simulink model "LCW_a"  (Simulink 8.7)
settings: Solver=ode1  SolverMode=SingleTasking  StartTime=0.0  StopTime=500  FixedStep=0.001  RelTol=1e-3
(part 3 of 4)

== system LCW_a/Veh_1/ComplexVehicleModel/Body and Tires/body_kinematic_out_whl_lf2 ==
  In1 : Inport
  Bus Creator : BusCreator  Inputs=18
  Demux : Demux  Outputs=18
  Out1 : Outport
  wires:
  In1/1 -> Demux/1
  Demux/1 -> Bus Creator/1  "rot_whl"
  Demux/2 -> Bus Creator/2  "w_whl"
  Demux/3 -> Bus Creator/3  "z_whl_whl"
  Demux/4 -> Bus Creator/4  "yaw_whl"
  Demux/5 -> Bus Creator/5  "pitch_whl"
  Demux/6 -> Bus Creator/6  "roll_whl"
  Demux/7 -> Bus Creator/7  "vwx_whl"
  Demux/8 -> Bus Creator/8  "vwy_whl"
  Demux/9 -> Bus Creator/9  "vwz_whl"
  Demux/10 -> Bus Creator/10  "avwx_whl"
  Demux/11 -> Bus Creator/11  "avwy_whl"
  Demux/12 -> Bus Creator/12  "avwz_whl"
  Demux/13 -> Bus Creator/13  "dzdx_whl"
  Demux/14 -> Bus Creator/14  "dzdy_whl"
  Demux/15 -> Bus Creator/15  "xgnd_whl"
  Demux/16 -> Bus Creator/16  "ygnd_whl"
  Demux/17 -> Bus Creator/17  "zgnd_whl"
  Demux/18 -> Bus Creator/18  "mux_whl"
  Bus Creator/1 -> Out1/1  "bodykin_whl_out"

== system LCW_a/Veh_1/ComplexVehicleModel/Body and Tires/body_kinematic_out_whl_lf3 ==
  In1 : Inport
  Bus Creator : BusCreator  Inputs=18
  Demux : Demux  Outputs=18
  Out1 : Outport
  wires:
  Bus Creator/1 -> Out1/1  "bodykin_whl_out"
  Demux/18 -> Bus Creator/18  "mux_whl"
  Demux/17 -> Bus Creator/17  "zgnd_whl"
  Demux/16 -> Bus Creator/16  "ygnd_whl"
  Demux/15 -> Bus Creator/15  "xgnd_whl"
  Demux/14 -> Bus Creator/14  "dzdy_whl"
  Demux/13 -> Bus Creator/13  "dzdx_whl"
  Demux/12 -> Bus Creator/12  "avwz_whl"
  Demux/11 -> Bus Creator/11  "avwy_whl"
  Demux/10 -> Bus Creator/10  "avwx_whl"
  Demux/9 -> Bus Creator/9  "vwz_whl"
  Demux/8 -> Bus Creator/8  "vwy_whl"
  Demux/7 -> Bus Creator/7  "vwx_whl"
  Demux/6 -> Bus Creator/6  "roll_whl"
  Demux/5 -> Bus Creator/5  "pitch_whl"
  Demux/4 -> Bus Creator/4  "yaw_whl"
  Demux/3 -> Bus Creator/3  "z_whl_whl"
  Demux/2 -> Bus Creator/2  "w_whl"
  Demux/1 -> Bus Creator/1  "rot_whl"
  In1/1 -> Demux/1

== system LCW_a/Veh_1/ComplexVehicleModel/Brake/Brake States ==
  In1 : Inport
  Bus Creator : BusCreator  Inputs=26
  Demux : Demux  Outputs=26
  Out1 : Outport
  wires:
  In1/1 -> Demux/1
  Demux/1 -> Bus Creator/1  "q0"
  Demux/2 -> Bus Creator/2  "q1"
  Demux/3 -> Bus Creator/3  "q2"
  Demux/4 -> Bus Creator/4  "q3"
  Demux/5 -> Bus Creator/5  "q4"
  Demux/6 -> Bus Creator/6  "q5"
  Demux/7 -> Bus Creator/7  "q6"
  Demux/8 -> Bus Creator/8  "q7"
  Demux/9 -> Bus Creator/9  "q8"
  Demux/10 -> Bus Creator/10  "q9"
  Demux/11 -> Bus Creator/11  "q10"
  Demux/12 -> Bus Creator/12  "q11"
  Demux/13 -> Bus Creator/13  "q12"
  Demux/14 -> Bus Creator/14  "u0"
  Demux/15 -> Bus Creator/15  "u1"
  Demux/16 -> Bus Creator/16  "u2"
  Bus Creator/1 -> Out1/1  "BrakeStates"
  Demux/17 -> Bus Creator/17  "u3"
  Demux/18 -> Bus Creator/18  "u4"
  Demux/19 -> Bus Creator/19  "u5"
  Demux/20 -> Bus Creator/20  "u6"
  Demux/21 -> Bus Creator/21  "u7"
  Demux/22 -> Bus Creator/22  "u8"
  Demux/23 -> Bus Creator/23  "u9"
  Demux/24 -> Bus Creator/24  "u10"
  Demux/25 -> Bus Creator/25  "u11"
  Demux/26 -> Bus Creator/26  "u12"

== system LCW_a/Veh_1/ComplexVehicleModel/Brake/SteerStates1 ==
  In1 : Inport
  Bus Creator : BusCreator  Inputs=22
  Demux : Demux  Outputs=22
  Out1 : Outport
  wires:
  Demux/22 -> Bus Creator/22  "turn_off"
  Demux/21 -> Bus Creator/21  "brake"
  Demux/20 -> Bus Creator/20  "trot_brk_rr"
  Demux/19 -> Bus Creator/19  "trot_brk_lr"
  Demux/18 -> Bus Creator/18  "trot_brk_rf"
  Demux/17 -> Bus Creator/17  "trot_brk_lf"
  Bus Creator/1 -> Out1/1  "BrakeOutput"
  Demux/16 -> Bus Creator/16  "mu_us_brk_rr"
  Demux/15 -> Bus Creator/15  "mu_us_brk_lr"
  Demux/14 -> Bus Creator/14  "mu_us_brk_rf"
  Demux/13 -> Bus Creator/13  "mu_us_brk_lf"
  Demux/12 -> Bus Creator/12  "fm_brk_rr"
  Demux/11 -> Bus Creator/11  "fm_brk_lr"
  Demux/10 -> Bus Creator/10  "fm_brk_rf"
  Demux/9 -> Bus Creator/9  "fm_brk_lf"
  Demux/8 -> Bus Creator/8  "pbkch_brk_rr"
  Demux/7 -> Bus Creator/7  "pbkch_brk_lr"
  Demux/6 -> Bus Creator/6  "pbkch_brk_rf"
  Demux/5 -> Bus Creator/5  "pbkch_brk_lf"
  Demux/4 -> Bus Creator/4  "fbk_out_brk"
  Demux/3 -> Bus Creator/3  "fbk_in_brk"
  Demux/2 -> Bus Creator/2  "fbk_pedal"
  Demux/1 -> Bus Creator/1  "pbk_con_brk"
  In1/1 -> Demux/1

== system LCW_a/Veh_1/ComplexVehicleModel/Powertrain/PowertrainOut ==
  In1 : Inport
  Bus Creator : BusCreator  Inputs=36
  Demux : Demux  Outputs=36
  Out1 : Outport
  wires:
  Bus Creator/1 -> Out1/1  "PowertrainOut"
  In1/1 -> Demux/1
  Demux/1 -> Bus Creator/1  "aa_eng"
  Demux/2 -> Bus Creator/2  "av_eng"
  Demux/3 -> Bus Creator/3  "av_eng_update"
  Demux/4 -> Bus Creator/4  "av_tc"
  Demux/5 -> Bus Creator/5  "fuel"
  Demux/6 -> Bus Creator/6  "iw_eff_pt_lf"
  Demux/7 -> Bus Creator/7  "iw_eff_pt_rf"
  Demux/8 -> Bus Creator/8  "iw_eff_pt_lr"
  Demux/9 -> Bus Creator/9  "iw_eff_pt_rr"
  Demux/10 -> Bus Creator/10  "my_drv_lf"
  Demux/11 -> Bus Creator/11  "my_drv_rf"
  Demux/12 -> Bus Creator/12  "my_drv_lr"
  Demux/13 -> Bus Creator/13  "my_drv_rr"
  Demux/14 -> Bus Creator/14  "pt_thr_eng"
  Demux/15 -> Bus Creator/15  "pt_throttle"
  Demux/16 -> Bus Creator/16  "pt_modetran"
  Demux/17 -> Bus Creator/17  "pt_rottrans"
  Demux/18 -> Bus Creator/18  "pt_m_engout"
  Demux/19 -> Bus Creator/19  "pt_m_eng_in"
  Demux/20 -> Bus Creator/20  "pt_gearauto"
  Demux/21 -> Bus Creator/21  "pt_gear_status"
  Demux/22 -> Bus Creator/22  "pt_gear_man"
  Demux/23 -> Bus Creator/23  "rot_eng_update"
  Demux/24 -> Bus Creator/24  "rot_tc"
  Demux/25 -> Bus Creator/25  "pt_av_trans"
  Demux/26 -> Bus Creator/26  "pt_m_tc"
  Demux/27 -> Bus Creator/27  "pt_m_trans"
  Demux/28 -> Bus Creator/28  "pt_pwrengin"
  Demux/29 -> Bus Creator/29  "pt_pwrengo"
  Demux/30 -> Bus Creator/30  "pt_pwrtrans"
  Demux/31 -> Bus Creator/31  "pt_pwrwheel"
  Demux/32 -> Bus Creator/32  "pt_pwr_tc"
  Demux/33 -> Bus Creator/33  "pt_clutch"
  Demux/34 -> Bus Creator/34  "pt_k_tc"
  Demux/35 -> Bus Creator/35  "pt_r_av_tc"
  Demux/36 -> Bus Creator/36  "pt_r_m_tc"

== system LCW_a/Veh_1/ComplexVehicleModel/Powertrain/PowertrainStates ==
  In1 : Inport
  Bus Creator : BusCreator  Inputs=38
  Demux : Demux  Outputs=38
  Out1 : Outport
  wires:
  In1/1 -> Demux/1
  Bus Creator/1 -> Out1/1  "PowertrainStates"
  Demux/1 -> Bus Creator/1  "q0"
  Demux/2 -> Bus Creator/2  "q1"
  Demux/3 -> Bus Creator/3  "q2"
  Demux/4 -> Bus Creator/4  "q3"
  Demux/5 -> Bus Creator/5  "q4"
  Demux/6 -> Bus Creator/6  "q5"
  Demux/7 -> Bus Creator/7  "q6"
  Demux/8 -> Bus Creator/8  "q7"
  Demux/9 -> Bus Creator/9  "q8"
  Demux/10 -> Bus Creator/10  "q9"
  Demux/11 -> Bus Creator/11  "q10"
  Demux/12 -> Bus Creator/12  "q11"
  Demux/13 -> Bus Creator/13  "q12"
  Demux/14 -> Bus Creator/14  "q13"
  Demux/15 -> Bus Creator/15  "q14"
  Demux/16 -> Bus Creator/16  "q15"
  Demux/17 -> Bus Creator/17  "q16"
  Demux/18 -> Bus Creator/18  "q17"
  Demux/19 -> Bus Creator/19  "q18"
  Demux/20 -> Bus Creator/20  "u0"
  Demux/21 -> Bus Creator/21  "u1"
  Demux/22 -> Bus Creator/22  "u2"
  Demux/23 -> Bus Creator/23  "u3"
  Demux/24 -> Bus Creator/24  "u4"
  Demux/25 -> Bus Creator/25  "u5"
  Demux/26 -> Bus Creator/26  "u6"
  Demux/27 -> Bus Creator/27  "u7"
  Demux/28 -> Bus Creator/28  "u8"
  Demux/29 -> Bus Creator/29  "u9"
  Demux/30 -> Bus Creator/30  "u10"
  Demux/31 -> Bus Creator/31  "u11"
  Demux/32 -> Bus Creator/32  "u12"
  Demux/33 -> Bus Creator/33  "u13"
  Demux/34 -> Bus Creator/34  "u14"
  Demux/35 -> Bus Creator/35  "u15"
  Demux/36 -> Bus Creator/36  "u16"
  Demux/37 -> Bus Creator/37  "u17"
  Demux/38 -> Bus Creator/38  "u18"

== system LCW_a/Veh_1/ComplexVehicleModel/Steer/SteerForces ==
  In1 : Inport
  Bus Creator : BusCreator  Inputs=32
  Demux : Demux  Outputs=32
  Out1 : Outport
  wires:
  Bus Creator/1 -> Out1/1  "Steer_Forces"
  Demux/26 -> Bus Creator/26  "steer_f_hys_2"
  Demux/25 -> Bus Creator/25  "steer_f_hys_1"
  Demux/24 -> Bus Creator/24  "steer_mkp_in_4"
  Demux/23 -> Bus Creator/23  "steer_mkp_in_3"
  Demux/22 -> Bus Creator/22  "steer_mkp_in_2"
  Demux/21 -> Bus Creator/21  "steer_mkp_in_1"
  Demux/20 -> Bus Creator/20  "steer_gear_dam_f_2"
  Demux/19 -> Bus Creator/19  "steer_boost_f_2"
  Demux/18 -> Bus Creator/18  "steer_gear_dam_t_2"
  Demux/17 -> Bus Creator/17  "steer_boost_t_2"
  Demux/16 -> Bus Creator/16  "steer_gear_dam_f_1"
  Demux/15 -> Bus Creator/15  "steer_boost_f_1"
  Demux/14 -> Bus Creator/14  "steer_gear_dam_t_1"
  Demux/13 -> Bus Creator/13  "steer_boost_t_1"
  Demux/12 -> Bus Creator/12  "steer_col_fric_t3"
  Demux/11 -> Bus Creator/11  "steer_col_dam_t3"
  Demux/10 -> Bus Creator/10  "steer_col_fric_t2"
  Demux/9 -> Bus Creator/9  "steer_col_dam_t2"
  Demux/8 -> Bus Creator/8  "steer_t_in1"
  Demux/7 -> Bus Creator/7  "steer_tbar_t1"
  Demux/6 -> Bus Creator/6  "steer_col_fric_t1"
  Demux/5 -> Bus Creator/5  "steer_col_dam_t1"
  Demux/4 -> Bus Creator/4  "steer_tbar_t"
  Demux/3 -> Bus Creator/3  "steer_col_fric_t"
  Demux/2 -> Bus Creator/2  "steer_col_dam_t"
  Demux/1 -> Bus Creator/1  "steer_t_in"
  In1/1 -> Demux/1
  Demux/27 -> Bus Creator/27  "steer_f_hys_3"
  Demux/28 -> Bus Creator/28  "steer_f_hys_4"
  Demux/29 -> Bus Creator/29  "m_kp_str_1"
  Demux/30 -> Bus Creator/30  "m_kp_str_2"
  Demux/31 -> Bus Creator/31  "m_kp_str_3"
  Demux/32 -> Bus Creator/32  "m_kp_str_4"

== system LCW_a/Veh_1/ComplexVehicleModel/Steer/SteerKinemateics ==
  In1 : Inport
  Bus Creator : BusCreator  Inputs=9
  Demux : Demux  Outputs=[4 1 1 1 1 4 4 4 2]
  Out1 : Outport
  wires:
  Bus Creator/1 -> Out1/1  "Steer_Kinematics"
  Demux/8 -> Bus Creator/8  "k_str"
  Demux/7 -> Bus Creator/7  "c_str"
  Demux/6 -> Bus Creator/6  "steer_str"
  Demux/5 -> Bus Creator/5  "str_sus_r"
  Demux/4 -> Bus Creator/4  "str_sus_f"
  Demux/3 -> Bus Creator/3  "strav_sw"
  Demux/2 -> Bus Creator/2  "drstr"
  Demux/1 -> Bus Creator/1  "str_whl_opt"
  In1/1 -> Demux/1
  Demux/9 -> Bus Creator/9  "strswr"

== system LCW_a/Veh_1/ComplexVehicleModel/Steer/SteerStates ==
  In1 : Inport
  Bus Creator : BusCreator  Inputs=26
  Demux : Demux  Outputs=26
  Out1 : Outport
  wires:
  In1/1 -> Demux/1
  Demux/1 -> Bus Creator/1  "q0"
  Demux/2 -> Bus Creator/2  "q1"
  Demux/3 -> Bus Creator/3  "q2"
  Demux/4 -> Bus Creator/4  "q3"
  Demux/5 -> Bus Creator/5  "q4"
  Demux/6 -> Bus Creator/6  "q5"
  Demux/7 -> Bus Creator/7  "q6"
  Demux/8 -> Bus Creator/8  "q7"
  Demux/9 -> Bus Creator/9  "q8"
  Demux/10 -> Bus Creator/10  "q9"
  Demux/11 -> Bus Creator/11  "q10"
  Demux/12 -> Bus Creator/12  "q11"
  Demux/13 -> Bus Creator/13  "q12"
  Demux/14 -> Bus Creator/14  "u0"
  Demux/15 -> Bus Creator/15  "u1"
  Demux/16 -> Bus Creator/16  "u2"
  Bus Creator/1 -> Out1/1  "SteerStates"
  Demux/17 -> Bus Creator/17  "u3"
  Demux/18 -> Bus Creator/18  "u4"
  Demux/19 -> Bus Creator/19  "u5"
  Demux/20 -> Bus Creator/20  "u6"
  Demux/21 -> Bus Creator/21  "u7"
  Demux/22 -> Bus Creator/22  "u8"
  Demux/23 -> Bus Creator/23  "u9"
  Demux/24 -> Bus Creator/24  "u10"
  Demux/25 -> Bus Creator/25  "u11"
  Demux/26 -> Bus Creator/26  "u12"

== system LCW_a/Veh_1/ComplexVehicleModel/Steer/SteerToBody ==
  In1 : Inport
  Bus Creator : BusCreator  Inputs=7
  Demux : Demux  Outputs=[2 4 4 4 4 4 4]
  Out1 : Outport
  wires:
  In1/1 -> Demux/1
  Demux/1 -> Bus Creator/1  "strratio"
  Demux/2 -> Bus Creator/2  "strc_str"
  Demux/3 -> Bus Creator/3  "kppc_str"
  Demux/4 -> Bus Creator/4  "kprc_str"
  Demux/5 -> Bus Creator/5  "rotd_kp_dr_str"
  Demux/6 -> Bus Creator/6  "rotd_kp_susp_str"
  Demux/7 -> Bus Creator/7  "gear_rotd_susp_str"
  Bus Creator/1 -> Out1/1  "Steer2Body"

== system LCW_a/Veh_1/ComplexVehicleModel/Suspensions/SupensionsStates ==
  In1 : Inport
  Bus Creator : BusCreator  Inputs=32
  Demux : Demux  Outputs=32
  Out1 : Outport
  wires:
  In1/1 -> Demux/1
  Demux/1 -> Bus Creator/1  "q0"
  Demux/2 -> Bus Creator/2  "q1"
  Demux/3 -> Bus Creator/3  "q2"
  Demux/4 -> Bus Creator/4  "q3"
  Demux/5 -> Bus Creator/5  "q4"
  Demux/6 -> Bus Creator/6  "q5"
  Demux/7 -> Bus Creator/7  "q6"
  Demux/8 -> Bus Creator/8  "q7"
  Demux/9 -> Bus Creator/9  "q8"
  Demux/10 -> Bus Creator/10  "q9"
  Demux/11 -> Bus Creator/11  "q10"
  Demux/12 -> Bus Creator/12  "q11"
  Demux/13 -> Bus Creator/13  "q12"
  Demux/14 -> Bus Creator/14  "q13"
  Demux/15 -> Bus Creator/15  "q14"
  Demux/16 -> Bus Creator/16  "q15"
  Bus Creator/1 -> Out1/1  "Suspensions States"
  Demux/17 -> Bus Creator/17  "u0"
  Demux/18 -> Bus Creator/18  "u1"
  Demux/19 -> Bus Creator/19  "u2"
  Demux/20 -> Bus Creator/20  "u3"
  Demux/21 -> Bus Creator/21  "u4"
  Demux/22 -> Bus Creator/22  "u5"
  Demux/23 -> Bus Creator/23  "u6"
  Demux/24 -> Bus Creator/24  "u7"
  Demux/25 -> Bus Creator/25  "u8"
  Demux/26 -> Bus Creator/26  "u9"
  Demux/27 -> Bus Creator/27  "u10"
  Demux/28 -> Bus Creator/28  "u11"
  Demux/29 -> Bus Creator/29  "u12"
  Demux/30 -> Bus Creator/30  "u13"
  Demux/31 -> Bus Creator/31  "u14"
  Demux/32 -> Bus Creator/32  "u15"

== system LCW_a/Veh_1/ComplexVehicleModel/Suspensions/SuspensionForces ==
  In1 : Inport
  Bus Creator : BusCreator  Inputs=18
  Demux : Demux  Outputs=18
  Out1 : Outport
  wires:
  Bus Creator/1 -> Out1/1  "SuspensionForces"
  In1/1 -> Demux/1
  Demux/1 -> Bus Creator/1  "spring_f_r1"
  Demux/2 -> Bus Creator/2  "spring_f_l1"
  Demux/3 -> Bus Creator/3  "spring_f_r2"
  Demux/4 -> Bus Creator/4  "spring_f_l2"
  Demux/5 -> Bus Creator/5  "jounce_stop_f_r1"
  Demux/6 -> Bus Creator/6  "reound_stop_f_r1"
  Demux/7 -> Bus Creator/7  "jounce_stop_f_l1"
  Demux/8 -> Bus Creator/8  "reound_stop_f_l1"
  Demux/9 -> Bus Creator/9  "jounce_stop_f_r2"
  Demux/10 -> Bus Creator/10  "reound_stop_f_r2"
  Demux/11 -> Bus Creator/11  "jounce_stop_f_l2"
  Demux/12 -> Bus Creator/12  "reound_stop_f_l2"
  Demux/13 -> Bus Creator/13  "damper_l1"
  Demux/14 -> Bus Creator/14  "damper_r1"
  Demux/15 -> Bus Creator/15  "damper_l2"
  Demux/16 -> Bus Creator/16  "damper_r2"
  Demux/17 -> Bus Creator/17  "maux_f"
  Demux/18 -> Bus Creator/18  "maux_r"

== system LCW_a/Veh_1/ComplexVehicleModel/Suspensions/SuspensionKinematics ==
  In1 : Inport
  Bus Creator : BusCreator  Inputs=23
  Demux : Demux  Outputs=[4 4 4 4 4 4 4 4 4 4 4 4 4 4 4 4 4 4 4 4 4 4 4]
  Out1 : Outport
  wires:
  Demux/23 -> Bus Creator/23  "fs_ext_susp"
  Demux/22 -> Bus Creator/22  "fs_susp"
  Demux/21 -> Bus Creator/21  "cmp_s_susp"
  Demux/20 -> Bus Creator/20  "cmprst_susp"
  Demux/19 -> Bus Creator/19  "cmprd_susp"
  Demux/18 -> Bus Creator/18  "cmpjst_susp"
  Demux/17 -> Bus Creator/17  "dcam_con_susp"
  Bus Creator/1 -> Out1/1  "SuspensionsKinematiocs"
  Demux/16 -> Bus Creator/16  "divedd_susp"
  Demux/15 -> Bus Creator/15  "dived_susp"
  Demux/14 -> Bus Creator/14  "dive_susp"
  Demux/13 -> Bus Creator/13  "toedd_susp"
  Demux/12 -> Bus Creator/12  "toed_susp"
  Demux/11 -> Bus Creator/11  "toe_susp"
  Demux/10 -> Bus Creator/10  "camdd_susp"
  Demux/9 -> Bus Creator/9  "camd_susp"
  Demux/8 -> Bus Creator/8  "cam_con_susp"
  Demux/7 -> Bus Creator/7  "cam_susp"
  Demux/6 -> Bus Creator/6  "latdd_susp"
  Demux/5 -> Bus Creator/5  "latd_susp"
  Demux/4 -> Bus Creator/4  "lat_susp"
  Demux/3 -> Bus Creator/3  "xdd_susp"
  Demux/2 -> Bus Creator/2  "xd_susp"
  Demux/1 -> Bus Creator/1  "x_susp"
  In1/1 -> Demux/1

== system LCW_a/Veh_1/ComplexVehicleModel/Suspensions/SuspensionSteer ==
  In1 : Inport
  Bus Creator : BusCreator  Inputs=3
  Demux : Demux  Outputs=[4 4 4]
  Out1 : Outport
  wires:
  Bus Creator/1 -> Out1/1  "SuspensionSteer"
  Demux/3 -> Bus Creator/3  "sw_mz_susp"
  Demux/2 -> Bus Creator/2  "sw_fy_susp"
  Demux/1 -> Bus Creator/1  "sw_fx_susp"
  In1/1 -> Demux/1

== system LCW_a/Veh_1/DriverModel/Driver/Driver2Brake ==
  In1 : Inport
  Bus Creator : BusCreator  Inputs=1
  Demux : Demux  Outputs=1
  Out1 : Outport
  wires:
  In1/1 -> Demux/1
  Demux/1 -> Bus Creator/1  "pcon_bk"
  Bus Creator/1 -> Out1/1  "Driver2Brake"

== system LCW_a/Veh_1/DriverModel/Driver/Driver2Powertrain ==
  In1 : Inport
  Bus Creator : BusCreator  Inputs=3
  Demux : Demux  Outputs=3
  Out1 : Outport
  wires:
  Bus Creator/1 -> Out1/1  "Driver2Powertrain"
  Demux/1 -> Bus Creator/1  "throttle"
  In1/1 -> Demux/1
  Demux/2 -> Bus Creator/2  "modetr"
  Demux/3 -> Bus Creator/3  "geartr"

== system LCW_a/Veh_1/DriverModel/Driver/Driver2Steer ==
  In1 : Inport
  Bus Creator : BusCreator  Inputs=1
  Demux : Demux  Outputs=1
  Out1 : Outport
  wires:
  In1/1 -> Demux/1
  Demux/1 -> Bus Creator/1  "drstr_drv"
  Bus Creator/1 -> Out1/1  "Driver2Steer"

== system LCW_a/Veh_1/DriverModel/Driver/DriverStates ==
  In1 : Inport
  Bus Creator : BusCreator  Inputs=4
  Demux : Demux
  Out1 : Outport
  wires:
  Bus Creator/1 -> Out1/1  "DriverStates"
  Demux/4 -> Bus Creator/4  "my_sc_r"
  Demux/3 -> Bus Creator/3  "my_sc_f"
  Demux/2 -> Bus Creator/2  "verr_drv"
  Demux/1 -> Bus Creator/1  "iverr_drv"
  In1/1 -> Demux/1

== system LCW_a/Veh_1_1/ComplexVehicleModel/Aerodynamics/Chassis States ==
  In1 : Inport
  Bus Creator : BusCreator  Inputs=12
  Demux : Demux  Outputs=12
  Out1 : Outport
  wires:
  In1/1 -> Demux/1
  Demux/1 -> Bus Creator/1  "beta_air"
  Demux/2 -> Bus Creator/2  "pitch_air"
  Demux/3 -> Bus Creator/3  "yawwind_air"
  Demux/4 -> Bus Creator/4  "v_air"
  Demux/5 -> Bus Creator/5  "vwind_air"
  Demux/6 -> Bus Creator/6  "z_air"
  Demux/7 -> Bus Creator/7  "fx_air"
  Demux/8 -> Bus Creator/8  "fy_air"
  Demux/9 -> Bus Creator/9  "fz_air"
  Demux/10 -> Bus Creator/10  "mx_air"
  Demux/11 -> Bus Creator/11  "my_air"
  Demux/12 -> Bus Creator/12  "mz_air"
  Bus Creator/1 -> Out1/1  "Aerodynamics_States"

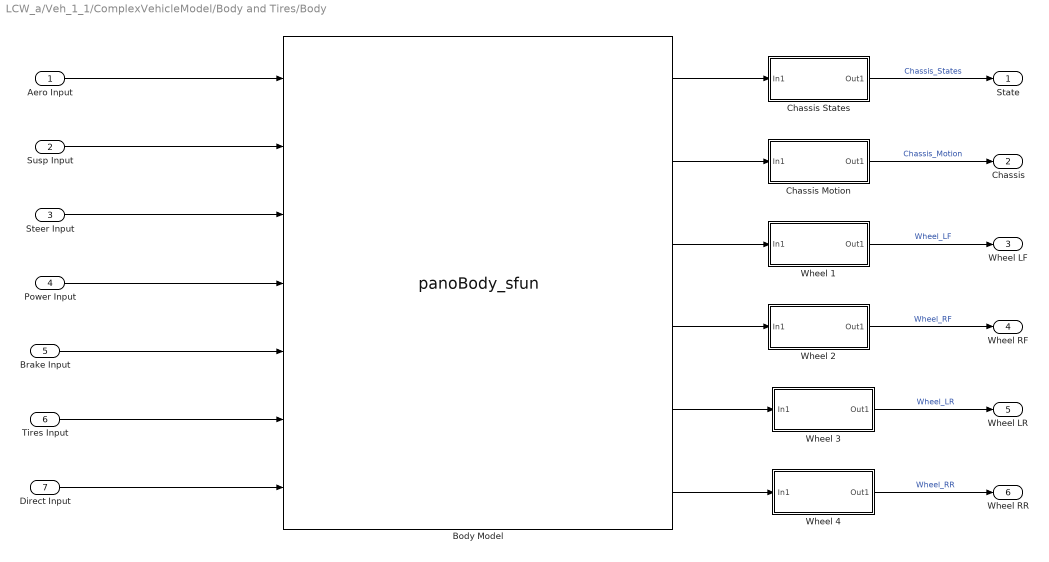
== system LCW_a/Veh_1_1/ComplexVehicleModel/Body and Tires/Body ==
  Aero Input : Inport
  Susp Input : Inport  Port=2
  Steer Input : Inport  Port=3
  Power Input : Inport  Port=4
  Brake Input : Inport  Port=5
  Tires Input : Inport  Port=6
  Direct Input : Inport  Port=7
  Body Model : S-Function  FunctionName=panoBody_sfun  Parameters='65ff4a6f-e423-428f-b9f1-c5e17da2fbba'  SFunctionDeploymentMode=off  EnableBusSupport=off
  Chassis Motion : Subsystem
  Chassis States : Subsystem
  Wheel 1 : Subsystem
  Wheel 2 : Subsystem
  Wheel 3 : Subsystem
  Wheel 4 : Subsystem
  State : Outport
  Chassis : Outport  Port=2
  Wheel LF : Outport  Port=3
  Wheel RF : Outport  Port=4
  Wheel LR : Outport  Port=5
  Wheel RR : Outport  Port=6
  wires:
  Direct Input/1 -> Body Model/7
  Body Model/2 -> Chassis Motion/1(In1)
  Chassis Motion/1(Out1) -> Chassis/1  "Chassis_Motion"
  Body Model/1 -> Chassis States/1(In1)
  Chassis States/1(Out1) -> State/1  "Chassis_States"
  Body Model/3 -> Wheel 1/1(In1)
  Wheel 1/1(Out1) -> Wheel LF/1  "Wheel_LF"
  Body Model/4 -> Wheel 2/1(In1)
  Body Model/5 -> Wheel 3/1(In1)
  Body Model/6 -> Wheel 4/1(In1)
  Wheel 3/1(Out1) -> Wheel LR/1  "Wheel_LR"
  Wheel 4/1(Out1) -> Wheel RR/1  "Wheel_RR"
  Wheel 2/1(Out1) -> Wheel RF/1  "Wheel_RF"
  Tires Input/1 -> Body Model/6
  Power Input/1 -> Body Model/4
  Brake Input/1 -> Body Model/5
  Steer Input/1 -> Body Model/3
  Susp Input/1 -> Body Model/2
  Aero Input/1 -> Body Model/1

== system LCW_a/Veh_1_1/ComplexVehicleModel/Body and Tires/Tires ==
  Wheel LF : Inport
  Wheel RF : Inport  Port=2
  Wheel LR : Inport  Port=3
  Wheel RR : Inport  Port=4
  Tires Force  2 : Subsystem
  "Tires Force 1 " : Subsystem
  Tires Force 3 : Subsystem
  Tires Force 4 : Subsystem
  Tires Force Ground : Subsystem
  Tires Model : S-Function  FunctionName=panoTire_sfun  Parameters='65ff4a6f-e423-428f-b9f1-c5e17da2fbba'  SFunctionDeploymentMode=off  EnableBusSupport=off
  TiresStates : Subsystem
  Tire States : Outport
  Tire LF : Outport  Port=2
  Tire RF : Outport  Port=3
  Tire LR : Outport  Port=4
  Tire RR : Outport  Port=5
  Tire Force Ground : Outport  Port=6
  wires:
  Tires Model/6 -> Tires Force Ground/1(In1)
  Tires Force Ground/1(Out1) -> Tire Force Ground/1  "Tire_Forces_GND"
  Wheel LF/1 -> Tires Model/1
  Wheel RF/1 -> Tires Model/2
  Wheel LR/1 -> Tires Model/3
  Wheel RR/1 -> Tires Model/4
  Tires Model/1 -> TiresStates/1(In1)
  TiresStates/1(Out1) -> Tire States/1  "Tires_States"
  Tires Model/2 -> "Tires Force 1 "/1(In1)
  "Tires Force 1 "/1(Out1) -> Tire LF/1  "Tire_Forces_LF"
  Tires Model/5 -> Tires Force 4/1(In1)
  Tires Model/4 -> Tires Force 3/1(In1)
  Tires Model/3 -> Tires Force  2/1(In1)
  Tires Force 3/1(Out1) -> Tire LR/1  "Tire_Forces_LR"
  Tires Force 4/1(Out1) -> Tire RR/1  "Tire_Forces_RR"
  Tires Force  2/1(Out1) -> Tire RF/1  "Tire_Forces_RF"

== system LCW_a/Veh_1_1/ComplexVehicleModel/Body and Tires/body_kinematic_out_whl_lf ==
  In1 : Inport
  Bus Creator : BusCreator  Inputs=18
  Demux : Demux  Outputs=18
  Out1 : Outport
  wires:
  In1/1 -> Demux/1
  Demux/1 -> Bus Creator/1  "rot_whl"
  Demux/2 -> Bus Creator/2  "w_whl"
  Demux/3 -> Bus Creator/3  "z_whl_whl"
  Demux/4 -> Bus Creator/4  "yaw_whl"
  Demux/5 -> Bus Creator/5  "pitch_whl"
  Demux/6 -> Bus Creator/6  "roll_whl"
  Demux/7 -> Bus Creator/7  "vwx_whl"
  Demux/8 -> Bus Creator/8  "vwy_whl"
  Demux/9 -> Bus Creator/9  "vwz_whl"
  Demux/10 -> Bus Creator/10  "avwx_whl"
  Demux/11 -> Bus Creator/11  "avwy_whl"
  Demux/12 -> Bus Creator/12  "avwz_whl"
  Demux/13 -> Bus Creator/13  "dzdx_whl"
  Demux/14 -> Bus Creator/14  "dzdy_whl"
  Demux/15 -> Bus Creator/15  "xgnd_whl"
  Demux/16 -> Bus Creator/16  "ygnd_whl"
  Demux/17 -> Bus Creator/17  "zgnd_whl"
  Demux/18 -> Bus Creator/18  "mux_whl"
  Bus Creator/1 -> Out1/1  "bodykin_whl_out"

== system LCW_a/Veh_1_1/ComplexVehicleModel/Body and Tires/body_kinematic_out_whl_lf1 ==
  In1 : Inport
  Bus Creator : BusCreator  Inputs=18
  Demux : Demux  Outputs=18
  Out1 : Outport
  wires:
  Bus Creator/1 -> Out1/1  "bodykin_whl_out"
  Demux/18 -> Bus Creator/18  "mux_whl"
  Demux/17 -> Bus Creator/17  "zgnd_whl"
  Demux/16 -> Bus Creator/16  "ygnd_whl"
  Demux/15 -> Bus Creator/15  "xgnd_whl"
  Demux/14 -> Bus Creator/14  "dzdy_whl"
  Demux/13 -> Bus Creator/13  "dzdx_whl"
  Demux/12 -> Bus Creator/12  "avwz_whl"
  Demux/11 -> Bus Creator/11  "avwy_whl"
  Demux/10 -> Bus Creator/10  "avwx_whl"
  Demux/9 -> Bus Creator/9  "vwz_whl"
  Demux/8 -> Bus Creator/8  "vwy_whl"
  Demux/7 -> Bus Creator/7  "vwx_whl"
  Demux/6 -> Bus Creator/6  "roll_whl"
  Demux/5 -> Bus Creator/5  "pitch_whl"
  Demux/4 -> Bus Creator/4  "yaw_whl"
  Demux/3 -> Bus Creator/3  "z_whl_whl"
  Demux/2 -> Bus Creator/2  "w_whl"
  Demux/1 -> Bus Creator/1  "rot_whl"
  In1/1 -> Demux/1

== system LCW_a/Veh_1_1/ComplexVehicleModel/Body and Tires/body_kinematic_out_whl_lf2 ==
  In1 : Inport
  Bus Creator : BusCreator  Inputs=18
  Demux : Demux  Outputs=18
  Out1 : Outport
  wires:
  In1/1 -> Demux/1
  Demux/1 -> Bus Creator/1  "rot_whl"
  Demux/2 -> Bus Creator/2  "w_whl"
  Demux/3 -> Bus Creator/3  "z_whl_whl"
  Demux/4 -> Bus Creator/4  "yaw_whl"
  Demux/5 -> Bus Creator/5  "pitch_whl"
  Demux/6 -> Bus Creator/6  "roll_whl"
  Demux/7 -> Bus Creator/7  "vwx_whl"
  Demux/8 -> Bus Creator/8  "vwy_whl"
  Demux/9 -> Bus Creator/9  "vwz_whl"
  Demux/10 -> Bus Creator/10  "avwx_whl"
  Demux/11 -> Bus Creator/11  "avwy_whl"
  Demux/12 -> Bus Creator/12  "avwz_whl"
  Demux/13 -> Bus Creator/13  "dzdx_whl"
  Demux/14 -> Bus Creator/14  "dzdy_whl"
  Demux/15 -> Bus Creator/15  "xgnd_whl"
  Demux/16 -> Bus Creator/16  "ygnd_whl"
  Demux/17 -> Bus Creator/17  "zgnd_whl"
  Demux/18 -> Bus Creator/18  "mux_whl"
  Bus Creator/1 -> Out1/1  "bodykin_whl_out"

== system LCW_a/Veh_1_1/ComplexVehicleModel/Body and Tires/body_kinematic_out_whl_lf3 ==
  In1 : Inport
  Bus Creator : BusCreator  Inputs=18
  Demux : Demux  Outputs=18
  Out1 : Outport
  wires:
  Bus Creator/1 -> Out1/1  "bodykin_whl_out"
  Demux/18 -> Bus Creator/18  "mux_whl"
  Demux/17 -> Bus Creator/17  "zgnd_whl"
  Demux/16 -> Bus Creator/16  "ygnd_whl"
  Demux/15 -> Bus Creator/15  "xgnd_whl"
  Demux/14 -> Bus Creator/14  "dzdy_whl"
  Demux/13 -> Bus Creator/13  "dzdx_whl"
  Demux/12 -> Bus Creator/12  "avwz_whl"
  Demux/11 -> Bus Creator/11  "avwy_whl"
  Demux/10 -> Bus Creator/10  "avwx_whl"
  Demux/9 -> Bus Creator/9  "vwz_whl"
  Demux/8 -> Bus Creator/8  "vwy_whl"
  Demux/7 -> Bus Creator/7  "vwx_whl"
  Demux/6 -> Bus Creator/6  "roll_whl"
  Demux/5 -> Bus Creator/5  "pitch_whl"
  Demux/4 -> Bus Creator/4  "yaw_whl"
  Demux/3 -> Bus Creator/3  "z_whl_whl"
  Demux/2 -> Bus Creator/2  "w_whl"
  Demux/1 -> Bus Creator/1  "rot_whl"
  In1/1 -> Demux/1

== system LCW_a/Veh_1_1/ComplexVehicleModel/Brake/Brake States ==
  In1 : Inport
  Bus Creator : BusCreator  Inputs=26
  Demux : Demux  Outputs=26
  Out1 : Outport
  wires:
  In1/1 -> Demux/1
  Demux/1 -> Bus Creator/1  "q0"
  Demux/2 -> Bus Creator/2  "q1"
  Demux/3 -> Bus Creator/3  "q2"
  Demux/4 -> Bus Creator/4  "q3"
  Demux/5 -> Bus Creator/5  "q4"
  Demux/6 -> Bus Creator/6  "q5"
  Demux/7 -> Bus Creator/7  "q6"
  Demux/8 -> Bus Creator/8  "q7"
  Demux/9 -> Bus Creator/9  "q8"
  Demux/10 -> Bus Creator/10  "q9"
  Demux/11 -> Bus Creator/11  "q10"
  Demux/12 -> Bus Creator/12  "q11"
  Demux/13 -> Bus Creator/13  "q12"
  Demux/14 -> Bus Creator/14  "u0"
  Demux/15 -> Bus Creator/15  "u1"
  Demux/16 -> Bus Creator/16  "u2"
  Bus Creator/1 -> Out1/1  "BrakeStates"
  Demux/17 -> Bus Creator/17  "u3"
  Demux/18 -> Bus Creator/18  "u4"
  Demux/19 -> Bus Creator/19  "u5"
  Demux/20 -> Bus Creator/20  "u6"
  Demux/21 -> Bus Creator/21  "u7"
  Demux/22 -> Bus Creator/22  "u8"
  Demux/23 -> Bus Creator/23  "u9"
  Demux/24 -> Bus Creator/24  "u10"
  Demux/25 -> Bus Creator/25  "u11"
  Demux/26 -> Bus Creator/26  "u12"

== system LCW_a/Veh_1_1/ComplexVehicleModel/Brake/SteerStates1 ==
  In1 : Inport
  Bus Creator : BusCreator  Inputs=22
  Demux : Demux  Outputs=22
  Out1 : Outport
  wires:
  Demux/22 -> Bus Creator/22  "turn_off"
  Demux/21 -> Bus Creator/21  "brake"
  Demux/20 -> Bus Creator/20  "trot_brk_rr"
  Demux/19 -> Bus Creator/19  "trot_brk_lr"
  Demux/18 -> Bus Creator/18  "trot_brk_rf"
  Demux/17 -> Bus Creator/17  "trot_brk_lf"
  Bus Creator/1 -> Out1/1  "BrakeOutput"
  Demux/16 -> Bus Creator/16  "mu_us_brk_rr"
  Demux/15 -> Bus Creator/15  "mu_us_brk_lr"
  Demux/14 -> Bus Creator/14  "mu_us_brk_rf"
  Demux/13 -> Bus Creator/13  "mu_us_brk_lf"
  Demux/12 -> Bus Creator/12  "fm_brk_rr"
  Demux/11 -> Bus Creator/11  "fm_brk_lr"
  Demux/10 -> Bus Creator/10  "fm_brk_rf"
  Demux/9 -> Bus Creator/9  "fm_brk_lf"
  Demux/8 -> Bus Creator/8  "pbkch_brk_rr"
  Demux/7 -> Bus Creator/7  "pbkch_brk_lr"
  Demux/6 -> Bus Creator/6  "pbkch_brk_rf"
  Demux/5 -> Bus Creator/5  "pbkch_brk_lf"
  Demux/4 -> Bus Creator/4  "fbk_out_brk"
  Demux/3 -> Bus Creator/3  "fbk_in_brk"
  Demux/2 -> Bus Creator/2  "fbk_pedal"
  Demux/1 -> Bus Creator/1  "pbk_con_brk"
  In1/1 -> Demux/1

== system LCW_a/Veh_1_1/ComplexVehicleModel/Powertrain/PowertrainOut ==
  In1 : Inport
  Bus Creator : BusCreator  Inputs=36
  Demux : Demux  Outputs=36
  Out1 : Outport
  wires:
  Bus Creator/1 -> Out1/1  "PowertrainOut"
  In1/1 -> Demux/1
  Demux/1 -> Bus Creator/1  "aa_eng"
  Demux/2 -> Bus Creator/2  "av_eng"
  Demux/3 -> Bus Creator/3  "av_eng_update"
  Demux/4 -> Bus Creator/4  "av_tc"
  Demux/5 -> Bus Creator/5  "fuel"
  Demux/6 -> Bus Creator/6  "iw_eff_pt_lf"
  Demux/7 -> Bus Creator/7  "iw_eff_pt_rf"
  Demux/8 -> Bus Creator/8  "iw_eff_pt_lr"
  Demux/9 -> Bus Creator/9  "iw_eff_pt_rr"
  Demux/10 -> Bus Creator/10  "my_drv_lf"
  Demux/11 -> Bus Creator/11  "my_drv_rf"
  Demux/12 -> Bus Creator/12  "my_drv_lr"
  Demux/13 -> Bus Creator/13  "my_drv_rr"
  Demux/14 -> Bus Creator/14  "pt_thr_eng"
  Demux/15 -> Bus Creator/15  "pt_throttle"
  Demux/16 -> Bus Creator/16  "pt_modetran"
  Demux/17 -> Bus Creator/17  "pt_rottrans"
  Demux/18 -> Bus Creator/18  "pt_m_engout"
  Demux/19 -> Bus Creator/19  "pt_m_eng_in"
  Demux/20 -> Bus Creator/20  "pt_gearauto"
  Demux/21 -> Bus Creator/21  "pt_gear_status"
  Demux/22 -> Bus Creator/22  "pt_gear_man"
  Demux/23 -> Bus Creator/23  "rot_eng_update"
  Demux/24 -> Bus Creator/24  "rot_tc"
  Demux/25 -> Bus Creator/25  "pt_av_trans"
  Demux/26 -> Bus Creator/26  "pt_m_tc"
  Demux/27 -> Bus Creator/27  "pt_m_trans"
  Demux/28 -> Bus Creator/28  "pt_pwrengin"
  Demux/29 -> Bus Creator/29  "pt_pwrengo"
  Demux/30 -> Bus Creator/30  "pt_pwrtrans"
  Demux/31 -> Bus Creator/31  "pt_pwrwheel"
  Demux/32 -> Bus Creator/32  "pt_pwr_tc"
  Demux/33 -> Bus Creator/33  "pt_clutch"
  Demux/34 -> Bus Creator/34  "pt_k_tc"
  Demux/35 -> Bus Creator/35  "pt_r_av_tc"
  Demux/36 -> Bus Creator/36  "pt_r_m_tc"

== system LCW_a/Veh_1_1/ComplexVehicleModel/Powertrain/PowertrainStates ==
  In1 : Inport
  Bus Creator : BusCreator  Inputs=38
  Demux : Demux  Outputs=38
  Out1 : Outport
  wires:
  In1/1 -> Demux/1
  Bus Creator/1 -> Out1/1  "PowertrainStates"
  Demux/1 -> Bus Creator/1  "q0"
  Demux/2 -> Bus Creator/2  "q1"
  Demux/3 -> Bus Creator/3  "q2"
  Demux/4 -> Bus Creator/4  "q3"
  Demux/5 -> Bus Creator/5  "q4"
  Demux/6 -> Bus Creator/6  "q5"
  Demux/7 -> Bus Creator/7  "q6"
  Demux/8 -> Bus Creator/8  "q7"
  Demux/9 -> Bus Creator/9  "q8"
  Demux/10 -> Bus Creator/10  "q9"
  Demux/11 -> Bus Creator/11  "q10"
  Demux/12 -> Bus Creator/12  "q11"
  Demux/13 -> Bus Creator/13  "q12"
  Demux/14 -> Bus Creator/14  "q13"
  Demux/15 -> Bus Creator/15  "q14"
  Demux/16 -> Bus Creator/16  "q15"
  Demux/17 -> Bus Creator/17  "q16"
  Demux/18 -> Bus Creator/18  "q17"
  Demux/19 -> Bus Creator/19  "q18"
  Demux/20 -> Bus Creator/20  "u0"
  Demux/21 -> Bus Creator/21  "u1"
  Demux/22 -> Bus Creator/22  "u2"
  Demux/23 -> Bus Creator/23  "u3"
  Demux/24 -> Bus Creator/24  "u4"
  Demux/25 -> Bus Creator/25  "u5"
  Demux/26 -> Bus Creator/26  "u6"
  Demux/27 -> Bus Creator/27  "u7"
  Demux/28 -> Bus Creator/28  "u8"
  Demux/29 -> Bus Creator/29  "u9"
  Demux/30 -> Bus Creator/30  "u10"
  Demux/31 -> Bus Creator/31  "u11"
  Demux/32 -> Bus Creator/32  "u12"
  Demux/33 -> Bus Creator/33  "u13"
  Demux/34 -> Bus Creator/34  "u14"
  Demux/35 -> Bus Creator/35  "u15"
  Demux/36 -> Bus Creator/36  "u16"
  Demux/37 -> Bus Creator/37  "u17"
  Demux/38 -> Bus Creator/38  "u18"

== system LCW_a/Veh_1_1/ComplexVehicleModel/Steer/SteerForces ==
  In1 : Inport
  Bus Creator : BusCreator  Inputs=32
  Demux : Demux  Outputs=32
  Out1 : Outport
  wires:
  Bus Creator/1 -> Out1/1  "Steer_Forces"
  Demux/26 -> Bus Creator/26  "steer_f_hys_2"
  Demux/25 -> Bus Creator/25  "steer_f_hys_1"
  Demux/24 -> Bus Creator/24  "steer_mkp_in_4"
  Demux/23 -> Bus Creator/23  "steer_mkp_in_3"
  Demux/22 -> Bus Creator/22  "steer_mkp_in_2"
  Demux/21 -> Bus Creator/21  "steer_mkp_in_1"
  Demux/20 -> Bus Creator/20  "steer_gear_dam_f_2"
  Demux/19 -> Bus Creator/19  "steer_boost_f_2"
  Demux/18 -> Bus Creator/18  "steer_gear_dam_t_2"
  Demux/17 -> Bus Creator/17  "steer_boost_t_2"
  Demux/16 -> Bus Creator/16  "steer_gear_dam_f_1"
  Demux/15 -> Bus Creator/15  "steer_boost_f_1"
  Demux/14 -> Bus Creator/14  "steer_gear_dam_t_1"
  Demux/13 -> Bus Creator/13  "steer_boost_t_1"
  Demux/12 -> Bus Creator/12  "steer_col_fric_t3"
  Demux/11 -> Bus Creator/11  "steer_col_dam_t3"
  Demux/10 -> Bus Creator/10  "steer_col_fric_t2"
  Demux/9 -> Bus Creator/9  "steer_col_dam_t2"
  Demux/8 -> Bus Creator/8  "steer_t_in1"
  Demux/7 -> Bus Creator/7  "steer_tbar_t1"
  Demux/6 -> Bus Creator/6  "steer_col_fric_t1"
  Demux/5 -> Bus Creator/5  "steer_col_dam_t1"
  Demux/4 -> Bus Creator/4  "steer_tbar_t"
  Demux/3 -> Bus Creator/3  "steer_col_fric_t"
  Demux/2 -> Bus Creator/2  "steer_col_dam_t"
  Demux/1 -> Bus Creator/1  "steer_t_in"
  In1/1 -> Demux/1
  Demux/27 -> Bus Creator/27  "steer_f_hys_3"
  Demux/28 -> Bus Creator/28  "steer_f_hys_4"
  Demux/29 -> Bus Creator/29  "m_kp_str_1"
  Demux/30 -> Bus Creator/30  "m_kp_str_2"
  Demux/31 -> Bus Creator/31  "m_kp_str_3"
  Demux/32 -> Bus Creator/32  "m_kp_str_4"

== system LCW_a/Veh_1_1/ComplexVehicleModel/Steer/SteerKinemateics ==
  In1 : Inport
  Bus Creator : BusCreator  Inputs=9
  Demux : Demux  Outputs=[4 1 1 1 1 4 4 4 2]
  Out1 : Outport
  wires:
  Bus Creator/1 -> Out1/1  "Steer_Kinematics"
  Demux/8 -> Bus Creator/8  "k_str"
  Demux/7 -> Bus Creator/7  "c_str"
  Demux/6 -> Bus Creator/6  "steer_str"
  Demux/5 -> Bus Creator/5  "str_sus_r"
  Demux/4 -> Bus Creator/4  "str_sus_f"
  Demux/3 -> Bus Creator/3  "strav_sw"
  Demux/2 -> Bus Creator/2  "drstr"
  Demux/1 -> Bus Creator/1  "str_whl_opt"
  In1/1 -> Demux/1
  Demux/9 -> Bus Creator/9  "strswr"

== system LCW_a/Veh_1_1/ComplexVehicleModel/Steer/SteerStates ==
  In1 : Inport
  Bus Creator : BusCreator  Inputs=26
  Demux : Demux  Outputs=26
  Out1 : Outport
  wires:
  In1/1 -> Demux/1
  Demux/1 -> Bus Creator/1  "q0"
  Demux/2 -> Bus Creator/2  "q1"
  Demux/3 -> Bus Creator/3  "q2"
  Demux/4 -> Bus Creator/4  "q3"
  Demux/5 -> Bus Creator/5  "q4"
  Demux/6 -> Bus Creator/6  "q5"
  Demux/7 -> Bus Creator/7  "q6"
  Demux/8 -> Bus Creator/8  "q7"
  Demux/9 -> Bus Creator/9  "q8"
  Demux/10 -> Bus Creator/10  "q9"
  Demux/11 -> Bus Creator/11  "q10"
  Demux/12 -> Bus Creator/12  "q11"
  Demux/13 -> Bus Creator/13  "q12"
  Demux/14 -> Bus Creator/14  "u0"
  Demux/15 -> Bus Creator/15  "u1"
  Demux/16 -> Bus Creator/16  "u2"
  Bus Creator/1 -> Out1/1  "SteerStates"
  Demux/17 -> Bus Creator/17  "u3"
  Demux/18 -> Bus Creator/18  "u4"
  Demux/19 -> Bus Creator/19  "u5"
  Demux/20 -> Bus Creator/20  "u6"
  Demux/21 -> Bus Creator/21  "u7"
  Demux/22 -> Bus Creator/22  "u8"
  Demux/23 -> Bus Creator/23  "u9"
  Demux/24 -> Bus Creator/24  "u10"
  Demux/25 -> Bus Creator/25  "u11"
  Demux/26 -> Bus Creator/26  "u12"

== system LCW_a/Veh_1_1/ComplexVehicleModel/Steer/SteerToBody ==
  In1 : Inport
  Bus Creator : BusCreator  Inputs=7
  Demux : Demux  Outputs=[2 4 4 4 4 4 4]
  Out1 : Outport
  wires:
  In1/1 -> Demux/1
  Demux/1 -> Bus Creator/1  "strratio"
  Demux/2 -> Bus Creator/2  "strc_str"
  Demux/3 -> Bus Creator/3  "kppc_str"
  Demux/4 -> Bus Creator/4  "kprc_str"
  Demux/5 -> Bus Creator/5  "rotd_kp_dr_str"
  Demux/6 -> Bus Creator/6  "rotd_kp_susp_str"
  Demux/7 -> Bus Creator/7  "gear_rotd_susp_str"
  Bus Creator/1 -> Out1/1  "Steer2Body"

== system LCW_a/Veh_1_1/ComplexVehicleModel/Suspensions/SupensionsStates ==
  In1 : Inport
  Bus Creator : BusCreator  Inputs=32
  Demux : Demux  Outputs=32
  Out1 : Outport
  wires:
  In1/1 -> Demux/1
  Demux/1 -> Bus Creator/1  "q0"
  Demux/2 -> Bus Creator/2  "q1"
  Demux/3 -> Bus Creator/3  "q2"
  Demux/4 -> Bus Creator/4  "q3"
  Demux/5 -> Bus Creator/5  "q4"
  Demux/6 -> Bus Creator/6  "q5"
  Demux/7 -> Bus Creator/7  "q6"
  Demux/8 -> Bus Creator/8  "q7"
  Demux/9 -> Bus Creator/9  "q8"
  Demux/10 -> Bus Creator/10  "q9"
  Demux/11 -> Bus Creator/11  "q10"
  Demux/12 -> Bus Creator/12  "q11"
  Demux/13 -> Bus Creator/13  "q12"
  Demux/14 -> Bus Creator/14  "q13"
  Demux/15 -> Bus Creator/15  "q14"
  Demux/16 -> Bus Creator/16  "q15"
  Bus Creator/1 -> Out1/1  "Suspensions States"
  Demux/17 -> Bus Creator/17  "u0"
  Demux/18 -> Bus Creator/18  "u1"
  Demux/19 -> Bus Creator/19  "u2"
  Demux/20 -> Bus Creator/20  "u3"
  Demux/21 -> Bus Creator/21  "u4"
  Demux/22 -> Bus Creator/22  "u5"
  Demux/23 -> Bus Creator/23  "u6"
  Demux/24 -> Bus Creator/24  "u7"
  Demux/25 -> Bus Creator/25  "u8"
  Demux/26 -> Bus Creator/26  "u9"
  Demux/27 -> Bus Creator/27  "u10"
  Demux/28 -> Bus Creator/28  "u11"
  Demux/29 -> Bus Creator/29  "u12"
  Demux/30 -> Bus Creator/30  "u13"
  Demux/31 -> Bus Creator/31  "u14"
  Demux/32 -> Bus Creator/32  "u15"

== system LCW_a/Veh_1_1/ComplexVehicleModel/Suspensions/SuspensionForces ==
  In1 : Inport
  Bus Creator : BusCreator  Inputs=18
  Demux : Demux  Outputs=18
  Out1 : Outport
  wires:
  Bus Creator/1 -> Out1/1  "SuspensionForces"
  In1/1 -> Demux/1
  Demux/1 -> Bus Creator/1  "spring_f_r1"
  Demux/2 -> Bus Creator/2  "spring_f_l1"
  Demux/3 -> Bus Creator/3  "spring_f_r2"
  Demux/4 -> Bus Creator/4  "spring_f_l2"
  Demux/5 -> Bus Creator/5  "jounce_stop_f_r1"
  Demux/6 -> Bus Creator/6  "reound_stop_f_r1"
  Demux/7 -> Bus Creator/7  "jounce_stop_f_l1"
  Demux/8 -> Bus Creator/8  "reound_stop_f_l1"
  Demux/9 -> Bus Creator/9  "jounce_stop_f_r2"
  Demux/10 -> Bus Creator/10  "reound_stop_f_r2"
  Demux/11 -> Bus Creator/11  "jounce_stop_f_l2"
  Demux/12 -> Bus Creator/12  "reound_stop_f_l2"
  Demux/13 -> Bus Creator/13  "damper_l1"
  Demux/14 -> Bus Creator/14  "damper_r1"
  Demux/15 -> Bus Creator/15  "damper_l2"
  Demux/16 -> Bus Creator/16  "damper_r2"
  Demux/17 -> Bus Creator/17  "maux_f"
  Demux/18 -> Bus Creator/18  "maux_r"

== system LCW_a/Veh_1_1/ComplexVehicleModel/Suspensions/SuspensionKinematics ==
  In1 : Inport
  Bus Creator : BusCreator  Inputs=23
  Demux : Demux  Outputs=[4 4 4 4 4 4 4 4 4 4 4 4 4 4 4 4 4 4 4 4 4 4 4]
  Out1 : Outport
  wires:
  Demux/23 -> Bus Creator/23  "fs_ext_susp"
  Demux/22 -> Bus Creator/22  "fs_susp"
  Demux/21 -> Bus Creator/21  "cmp_s_susp"
  Demux/20 -> Bus Creator/20  "cmprst_susp"
  Demux/19 -> Bus Creator/19  "cmprd_susp"
  Demux/18 -> Bus Creator/18  "cmpjst_susp"
  Demux/17 -> Bus Creator/17  "dcam_con_susp"
  Bus Creator/1 -> Out1/1  "SuspensionsKinematiocs"
  Demux/16 -> Bus Creator/16  "divedd_susp"
  Demux/15 -> Bus Creator/15  "dived_susp"
  Demux/14 -> Bus Creator/14  "dive_susp"
  Demux/13 -> Bus Creator/13  "toedd_susp"
  Demux/12 -> Bus Creator/12  "toed_susp"
  Demux/11 -> Bus Creator/11  "toe_susp"
  Demux/10 -> Bus Creator/10  "camdd_susp"
  Demux/9 -> Bus Creator/9  "camd_susp"
  Demux/8 -> Bus Creator/8  "cam_con_susp"
  Demux/7 -> Bus Creator/7  "cam_susp"
  Demux/6 -> Bus Creator/6  "latdd_susp"
  Demux/5 -> Bus Creator/5  "latd_susp"
  Demux/4 -> Bus Creator/4  "lat_susp"
  Demux/3 -> Bus Creator/3  "xdd_susp"
  Demux/2 -> Bus Creator/2  "xd_susp"
  Demux/1 -> Bus Creator/1  "x_susp"
  In1/1 -> Demux/1

== system LCW_a/Veh_1_1/ComplexVehicleModel/Suspensions/SuspensionSteer ==
  In1 : Inport
  Bus Creator : BusCreator  Inputs=3
  Demux : Demux  Outputs=[4 4 4]
  Out1 : Outport
  wires:
  Bus Creator/1 -> Out1/1  "SuspensionSteer"
  Demux/3 -> Bus Creator/3  "sw_mz_susp"
  Demux/2 -> Bus Creator/2  "sw_fy_susp"
  Demux/1 -> Bus Creator/1  "sw_fx_susp"
  In1/1 -> Demux/1

== system LCW_a/Veh_1_1/DriverModel/Driver/Driver2Brake ==
  In1 : Inport
  Bus Creator : BusCreator  Inputs=1
  Demux : Demux  Outputs=1
  Out1 : Outport
  wires:
  In1/1 -> Demux/1
  Demux/1 -> Bus Creator/1  "pcon_bk"
  Bus Creator/1 -> Out1/1  "Driver2Brake"

== system LCW_a/Veh_1_1/DriverModel/Driver/Driver2Powertrain ==
  In1 : Inport
  Bus Creator : BusCreator  Inputs=3
  Demux : Demux  Outputs=3
  Out1 : Outport
  wires:
  Bus Creator/1 -> Out1/1  "Driver2Powertrain"
  Demux/1 -> Bus Creator/1  "throttle"
  In1/1 -> Demux/1
  Demux/2 -> Bus Creator/2  "modetr"
  Demux/3 -> Bus Creator/3  "geartr"

== system LCW_a/Veh_1_1/DriverModel/Driver/Driver2Steer ==
  In1 : Inport
  Bus Creator : BusCreator  Inputs=1
  Demux : Demux  Outputs=1
  Out1 : Outport
  wires:
  In1/1 -> Demux/1
  Demux/1 -> Bus Creator/1  "drstr_drv"
  Bus Creator/1 -> Out1/1  "Driver2Steer"

== system LCW_a/Veh_1_1/DriverModel/Driver/DriverStates ==
  In1 : Inport
  Bus Creator : BusCreator  Inputs=4
  Demux : Demux
  Out1 : Outport
  wires:
  Bus Creator/1 -> Out1/1  "DriverStates"
  Demux/4 -> Bus Creator/4  "my_sc_r"
  Demux/3 -> Bus Creator/3  "my_sc_f"
  Demux/2 -> Bus Creator/2  "verr_drv"
  Demux/1 -> Bus Creator/1  "iverr_drv"
  In1/1 -> Demux/1

== system LCW_a/Veh_1/ComplexVehicleModel/Body and Tires/Body/Chassis Motion ==
  In1 : Inport
  Bus Creator : BusCreator  Inputs=54
  Demux : Demux  Outputs=54
  Out1 : Outport
  wires:
  Bus Creator/1 -> Out1/1
  Demux/54 -> Bus Creator/54  "ZO"
  Demux/53 -> Bus Creator/53  "ZCG_TM"
  Demux/52 -> Bus Creator/52  "ZCG_SM"
  Demux/51 -> Bus Creator/51  "YO"
  Demux/50 -> Bus Creator/50  "YCG_TM"
  Demux/49 -> Bus Creator/49  "YCG_SM"
  Demux/48 -> Bus Creator/48  "YAW"
  Demux/47 -> Bus Creator/47  "XO"
  Demux/46 -> Bus Creator/46  "XCG_TM"
  Demux/45 -> Bus Creator/45  "XCG_SM"
  Demux/44 -> Bus Creator/44  "VZ_SM"
  Demux/43 -> Bus Creator/43  "VZBF_SM"
  Demux/42 -> Bus Creator/42  "VZ"
  Demux/41 -> Bus Creator/41  "VY_SM"
  Demux/40 -> Bus Creator/40  "VYNF_SM"
  Demux/39 -> Bus Creator/39  "VYBF_SM"
  Demux/38 -> Bus Creator/38  "VY"
  Demux/37 -> Bus Creator/37  "VX_SM"
  Demux/36 -> Bus Creator/36  "VXNF_SM"
  Demux/35 -> Bus Creator/35  "VXBF_SM"
  Demux/34 -> Bus Creator/34  "VX"
  Demux/33 -> Bus Creator/33  "ROLL_E"
  Demux/32 -> Bus Creator/32  "ROLL"
  Demux/31 -> Bus Creator/31  "PITCH"
  Demux/30 -> Bus Creator/30  "KUG_STRR"
  Demux/29 -> Bus Creator/29  "KUG_GND"
  Demux/28 -> Bus Creator/28  "KSF_STRR"
  Demux/27 -> Bus Creator/27  "KSF_GND"
  Demux/26 -> Bus Creator/26  "BETAR"
  Demux/25 -> Bus Creator/25  "BETA"
  Demux/24 -> Bus Creator/24  "AZ_SM"
  Demux/23 -> Bus Creator/23  "AZBF_SM"
  Demux/22 -> Bus Creator/22  "AZ"
  Demux/21 -> Bus Creator/21  "AY_SM"
  Demux/20 -> Bus Creator/20  "AYNF_SM"
  Demux/19 -> Bus Creator/19  "AYG_SM"
  Demux/18 -> Bus Creator/18  "AYBF_SM"
  Demux/17 -> Bus Creator/17  "AY"
  Demux/16 -> Bus Creator/16  "AX_SM"
  Demux/15 -> Bus Creator/15  "AXNF_SM"
  Demux/14 -> Bus Creator/14  "AXBF_SM"
  Demux/13 -> Bus Creator/13  "AX"
  Demux/12 -> Bus Creator/12  "AV_Y"
  Demux/11 -> Bus Creator/11  "AV_R"
  Demux/10 -> Bus Creator/10  "AV_P"
  Demux/9 -> Bus Creator/9  "AVZ"
  Demux/8 -> Bus Creator/8  "AVY"
  Demux/7 -> Bus Creator/7  "AVX"
  Demux/6 -> Bus Creator/6  "AA_Y"
  Demux/5 -> Bus Creator/5  "AA_R"
  Demux/4 -> Bus Creator/4  "AA_P"
  Demux/3 -> Bus Creator/3  "AAZ"
  Demux/2 -> Bus Creator/2  "AAY"
  Demux/1 -> Bus Creator/1  "AAX"
  In1/1 -> Demux/1

== system LCW_a/Veh_1/ComplexVehicleModel/Body and Tires/Body/Chassis States ==
  In1 : Inport
  Bus Creator : BusCreator  Inputs=24
  Demux : Demux  Outputs=24
  Out1 : Outport
  wires:
  In1/1 -> Demux/1
  Demux/1 -> Bus Creator/1  "q0"
  Demux/2 -> Bus Creator/2  "q1"
  Demux/3 -> Bus Creator/3  "q2"
  Demux/4 -> Bus Creator/4  "q3"
  Demux/5 -> Bus Creator/5  "q4"
  Demux/6 -> Bus Creator/6  "q5"
  Demux/7 -> Bus Creator/7  "q6"
  Demux/8 -> Bus Creator/8  "q7"
  Demux/9 -> Bus Creator/9  "u0"
  Demux/10 -> Bus Creator/10  "u1"
  Demux/11 -> Bus Creator/11  "u2"
  Demux/12 -> Bus Creator/12  "u3"
  Demux/13 -> Bus Creator/13  "u4"
  Demux/14 -> Bus Creator/14  "u5"
  Demux/15 -> Bus Creator/15  "u6"
  Demux/16 -> Bus Creator/16  "u7"
  Bus Creator/1 -> Out1/1  "Chassis States"
  Demux/17 -> Bus Creator/17  "up0"
  Demux/18 -> Bus Creator/18  "up1"
  Demux/19 -> Bus Creator/19  "up2"
  Demux/20 -> Bus Creator/20  "up3"
  Demux/21 -> Bus Creator/21  "up4"
  Demux/22 -> Bus Creator/22  "up5"
  Demux/23 -> Bus Creator/23  "up6"
  Demux/24 -> Bus Creator/24  "up7"

== system LCW_a/Veh_1/ComplexVehicleModel/Body and Tires/Body/Wheel 1 ==
  In1 : Inport
  Bus Creator : BusCreator  Inputs=13
  Demux : Demux  Outputs=13
  Out1 : Outport
  wires:
  Bus Creator/1 -> Out1/1
  Demux/8 -> Bus Creator/8  "fy_whl"
  Demux/7 -> Bus Creator/7  "fx_whl"
  Demux/5 -> Bus Creator/5  "up0"
  Demux/4 -> Bus Creator/4  "u1"
  Demux/3 -> Bus Creator/3  "u0"
  Demux/2 -> Bus Creator/2  "q1"
  Demux/1 -> Bus Creator/1  "q0"
  In1/1 -> Demux/1
  Demux/6 -> Bus Creator/6  "up1"
  Demux/13 -> Bus Creator/13  "h_wc"
  Demux/12 -> Bus Creator/12  "mz_whl"
  Demux/11 -> Bus Creator/11  "my_whl"
  Demux/10 -> Bus Creator/10  "mx_whl"
  Demux/9 -> Bus Creator/9  "fz_whl"

== system LCW_a/Veh_1/ComplexVehicleModel/Body and Tires/Body/Wheel 2 ==
  In1 : Inport
  Bus Creator : BusCreator  Inputs=13
  Demux : Demux  Outputs=13
  Out1 : Outport
  wires:
  Bus Creator/1 -> Out1/1
  Demux/8 -> Bus Creator/8  "fy_whl"
  Demux/7 -> Bus Creator/7  "fx_whl"
  Demux/5 -> Bus Creator/5  "up0"
  Demux/4 -> Bus Creator/4  "u1"
  Demux/3 -> Bus Creator/3  "u0"
  Demux/2 -> Bus Creator/2  "q1"
  Demux/1 -> Bus Creator/1  "q0"
  In1/1 -> Demux/1
  Demux/6 -> Bus Creator/6  "up1"
  Demux/13 -> Bus Creator/13  "h_wc"
  Demux/12 -> Bus Creator/12  "mz_whl"
  Demux/11 -> Bus Creator/11  "my_whl"
  Demux/10 -> Bus Creator/10  "mx_whl"
  Demux/9 -> Bus Creator/9  "fz_whl"

== system LCW_a/Veh_1/ComplexVehicleModel/Body and Tires/Body/Wheel 3 ==
  In1 : Inport
  Bus Creator : BusCreator  Inputs=13
  Demux : Demux  Outputs=13
  Out1 : Outport
  wires:
  Bus Creator/1 -> Out1/1
  Demux/8 -> Bus Creator/8  "fy_whl"
  Demux/7 -> Bus Creator/7  "fx_whl"
  Demux/5 -> Bus Creator/5  "up0"
  Demux/4 -> Bus Creator/4  "u1"
  Demux/3 -> Bus Creator/3  "u0"
  Demux/2 -> Bus Creator/2  "q1"
  Demux/1 -> Bus Creator/1  "q0"
  In1/1 -> Demux/1
  Demux/6 -> Bus Creator/6  "up1"
  Demux/13 -> Bus Creator/13  "h_wc"
  Demux/12 -> Bus Creator/12  "mz_whl"
  Demux/11 -> Bus Creator/11  "my_whl"
  Demux/10 -> Bus Creator/10  "mx_whl"
  Demux/9 -> Bus Creator/9  "fz_whl"

== system LCW_a/Veh_1/ComplexVehicleModel/Body and Tires/Body/Wheel 4 ==
  In1 : Inport
  Bus Creator : BusCreator  Inputs=13
  Demux : Demux  Outputs=13
  Out1 : Outport
  wires:
  Bus Creator/1 -> Out1/1
  Demux/8 -> Bus Creator/8  "fy_whl"
  Demux/7 -> Bus Creator/7  "fx_whl"
  Demux/5 -> Bus Creator/5  "up0"
  Demux/4 -> Bus Creator/4  "u1"
  Demux/3 -> Bus Creator/3  "u0"
  Demux/2 -> Bus Creator/2  "q1"
  Demux/1 -> Bus Creator/1  "q0"
  In1/1 -> Demux/1
  Demux/6 -> Bus Creator/6  "up1"
  Demux/13 -> Bus Creator/13  "h_wc"
  Demux/12 -> Bus Creator/12  "mz_whl"
  Demux/11 -> Bus Creator/11  "my_whl"
  Demux/10 -> Bus Creator/10  "mx_whl"
  Demux/9 -> Bus Creator/9  "fz_whl"

== system LCW_a/Veh_1/ComplexVehicleModel/Body and Tires/Tires/Tires Force  2 ==
  In1 : Inport
  Bus Creator : BusCreator  Inputs=6
  Demux : Demux  Outputs=6
  Out1 : Outport
  wires:
  Bus Creator/1 -> Out1/1  "Tires_Forces"
  Demux/6 -> Bus Creator/6  "mz"
  Demux/5 -> Bus Creator/5  "my"
  Demux/4 -> Bus Creator/4  "mx"
  Demux/3 -> Bus Creator/3  "fz"
  In1/1 -> Demux/1
  Demux/2 -> Bus Creator/2  "fy"
  Demux/1 -> Bus Creator/1  "fx"

== system LCW_a/Veh_1/ComplexVehicleModel/Body and Tires/Tires/Tires Force 1  ==
  In1 : Inport
  Bus Creator : BusCreator  Inputs=6
  Demux : Demux  Outputs=6
  Out1 : Outport
  wires:
  Demux/1 -> Bus Creator/1  "fx"
  Demux/2 -> Bus Creator/2  "fy"
  In1/1 -> Demux/1
  Demux/3 -> Bus Creator/3  "fz"
  Demux/4 -> Bus Creator/4  "mx"
  Demux/5 -> Bus Creator/5  "my"
  Demux/6 -> Bus Creator/6  "mz"
  Bus Creator/1 -> Out1/1  "Tires_Forces"

== system LCW_a/Veh_1/ComplexVehicleModel/Body and Tires/Tires/Tires Force 3 ==
  In1 : Inport
  Bus Creator : BusCreator  Inputs=6
  Demux : Demux  Outputs=6
  Out1 : Outport
  wires:
  Demux/1 -> Bus Creator/1  "fx"
  Demux/2 -> Bus Creator/2  "fy"
  In1/1 -> Demux/1
  Demux/3 -> Bus Creator/3  "fz"
  Demux/4 -> Bus Creator/4  "mx"
  Demux/5 -> Bus Creator/5  "my"
  Demux/6 -> Bus Creator/6  "mz"
  Bus Creator/1 -> Out1/1  "Tires_Forces"

== system LCW_a/Veh_1/ComplexVehicleModel/Body and Tires/Tires/Tires Force 4 ==
  In1 : Inport
  Bus Creator : BusCreator  Inputs=6
  Demux : Demux  Outputs=6
  Out1 : Outport
  wires:
  Bus Creator/1 -> Out1/1  "Tires_Forces"
  Demux/6 -> Bus Creator/6  "mz"
  Demux/5 -> Bus Creator/5  "my"
  Demux/4 -> Bus Creator/4  "mx"
  Demux/3 -> Bus Creator/3  "fz"
  In1/1 -> Demux/1
  Demux/2 -> Bus Creator/2  "fy"
  Demux/1 -> Bus Creator/1  "fx"

== system LCW_a/Veh_1/ComplexVehicleModel/Body and Tires/Tires/Tires Force Ground ==
  In1 : Inport
  Bus Creator : BusCreator  Inputs=24
  Demux : Demux  Outputs=24
  Out1 : Outport
  wires:
  Demux/24 -> Bus Creator/24  "mz_gnd_r2"
  Demux/23 -> Bus Creator/23  "my_gnd_r2"
  Demux/22 -> Bus Creator/22  "mx_gnd_r2"
  Demux/21 -> Bus Creator/21  "fz_gnd_r2"
  Demux/20 -> Bus Creator/20  "fy_gnd_r2"
  Demux/19 -> Bus Creator/19  "fx_gnd_r2"
  Demux/18 -> Bus Creator/18  "mz_gnd_l2"
  Demux/17 -> Bus Creator/17  "my_gnd_l2"
  Demux/16 -> Bus Creator/16  "mx_gnd_l2"
  Demux/15 -> Bus Creator/15  "fz_gnd_l2"
  Demux/14 -> Bus Creator/14  "fy_gnd_l2"
  Demux/13 -> Bus Creator/13  "fx_gnd_l2"
  Demux/12 -> Bus Creator/12  "mz_gnd_r1"
  Demux/11 -> Bus Creator/11  "my_gnd_r1"
  Demux/10 -> Bus Creator/10  "mx_gnd_r1"
  Demux/9 -> Bus Creator/9  "fz_gnd_r1"
  Demux/8 -> Bus Creator/8  "fy_gnd_r1"
  Demux/7 -> Bus Creator/7  "fx_gnd_r1"
  Demux/1 -> Bus Creator/1  "fx_gnd_l1"
  Demux/2 -> Bus Creator/2  "fy_gnd_l1"
  In1/1 -> Demux/1
  Demux/3 -> Bus Creator/3  "fz_gnd_l1"
  Demux/4 -> Bus Creator/4  "mx_gnd_l1"
  Demux/5 -> Bus Creator/5  "my_gnd_l1"
  Demux/6 -> Bus Creator/6  "mz_gnd_l1"
  Bus Creator/1 -> Out1/1  "Tires_Forces"

== system LCW_a/Veh_1/ComplexVehicleModel/Body and Tires/Tires/TiresStates ==
  In1 : Inport
  Bus Creator : BusCreator  Inputs=16
  Demux : Demux  Outputs=16
  Out1 : Outport
  wires:
  In1/1 -> Demux/1
  Demux/1 -> Bus Creator/1  "slip_lat_lf"
  Demux/2 -> Bus Creator/2  "slip_long_lf"
  Demux/3 -> Bus Creator/3  "slip_lat_rf"
  Demux/4 -> Bus Creator/4  "slip_long_rf"
  Demux/5 -> Bus Creator/5  "slip_lat_lr"
  Demux/6 -> Bus Creator/6  "slip_long_lr"
  Demux/7 -> Bus Creator/7  "slip_lat_rr"
  Demux/8 -> Bus Creator/8  "slip_long_rr"
  Demux/9 -> Bus Creator/9  "dslip_lat_lf"
  Demux/10 -> Bus Creator/10  "dslip_long_lf"
  Demux/11 -> Bus Creator/11  "dslip_lat_rf"
  Demux/12 -> Bus Creator/12  "dslip_long_rf"
  Demux/13 -> Bus Creator/13  "dslip_lat_lr"
  Demux/14 -> Bus Creator/14  "dslip_long_lr"
  Demux/15 -> Bus Creator/15  "dslip_lat_rr"
  Demux/16 -> Bus Creator/16  "dslip_long_rr"
  Bus Creator/1 -> Out1/1  "Tires_States"
